simulink model "chap6_4sim"  (Simulink 5.0)
settings: Solver=ode45  StartTime=0.0  StopTime=2  FixedStep=0.001  RelTol=1e-3
settings Model: LastModifiedBy=Administrator  ExtModeTrigMode=oneshot  ExtModeArmWhenConnect=off  LimitDataPoints=off  BooleanDataType=off

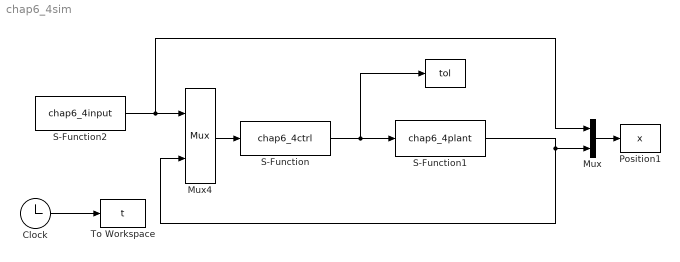
== system chap6_4sim ==
  "  " : ToWorkspace  VariableName=tol  SampleTime=-1  SaveFormat=Array
  Clock : Clock
      settings: Decimation=10
  Mux : Mux  Inputs=2
  Mux4 : Mux  Inputs=2
  Position1 : ToWorkspace  VariableName=x  SampleTime=-1  SaveFormat=Array
  S-Function : S-Function  FunctionName=chap6_4ctrl
  S-Function1 : S-Function  FunctionName=chap6_4plant
  S-Function2 : S-Function  FunctionName=chap6_4input
  To Workspace : ToWorkspace  VariableName=t  SampleTime=-1  SaveFormat=Array
  wires:
  S-Function/1 -> S-Function1/1, "  "/1
  S-Function1/1 -> Mux4/2, Mux/2
  Clock/1 -> To Workspace/1
  Mux4/1 -> S-Function/1
  S-Function2/1 -> Mux4/1, Mux/1
  Mux/1 -> Position1/1
